simulink model "CSI_0313_4DC"  (R2018a)
settings: Solver=FixedStepDiscrete  StartTime=0.0  StopTime=Tstop  FixedStep=Tdelt  MaxStep=1e-4  RelTol=1e-3
values from neighbouring files (symbols this model uses):
  C = 12e-6    (= 1.2e-05)    [Inputparameter.m]
  Cdc = 4.76*10^-3    (= 0.00476)    [Inputparameter.m]
  Cemc = 1.5e-6    (= 1.5e-06)    [Inputparameter.m]
  fanalog = 7000    [Run.m]
  fKIUdc = 6    [Run.m]
  fKPUdc = 0.4    [Run.m]
  fTs = Update/18000    (= 0.000111111111111)    [Run.m]
  K120 = 0.0    (= 0)    [Run.m]
  K21 = 0.0    (= 0)    [Run.m]
  K5 = 0.0    (= 0)    [Run.m]
  K7 = 0.0    (= 0)    [Run.m]
  Kipll = 1.0    (= 1)    [Run.m]
  klmt = 0.3    [Run.m]
  Kpll = 20.0    (= 20)    [Run.m]
  Lgrid = 7.717e-4*10    (= 0.007717)    [Run.m]
  Lline = 60e-6    (= 6e-05)    [Inputparameter.m]
  Lpwm = 184.8e-6    (= 0.0001848)    [Inputparameter.m]
  mode = 1    [Run.m]
  Nsw = 18000/fbase    [Run.m]
  Qbpf = 1.0    (= 1)    [Run.m]
  Rc = 10e-3    (= 0.01)    [Inputparameter.m]
  Remc = 1e-3    (= 0.001)    [Inputparameter.m]
  Rgrid = 2*pi*fbase*Lgrid/XR    [Run.m]
  Rline = 4.95e-3    (= 0.00495)    [Inputparameter.m]
  Rpre = 2.2    [Inputparameter.m]
  Rpwm = 6.2e-3    (= 0.0062)    [Inputparameter.m]
  Tdelt = (fTs)/(200*Update)    (= 2.77777777778e-07)    [Run.m]
  Tdt = 1.27e-6    (= 1.27e-06)    [Run.m]
  tstart = 0.2    [Run.m]
  Tvstep = 1.5    [Run.m]
  Update = 2    [Run.m]
  Vbase = 400*sqrt(2/3)    [Inputparameter.m]
undefined symbols (not defined in the file or in its folder): sigbuilder_block
libraries: powerlib x412
(part 12 of 13)

== matlab function CSI_0313_4DC/AIP6/Subsystem5/PLL/Pos&Neg seq extract in subsystem /IIR_BPF_Re1 ==
  data: u input; fn input; fQ parameter; y output; fTs parameter; iMode parameter
function y =IIR_2rd(u, fn, fQ, fTs, iMode)
    % Second order transfer function used for LPF and BPF
    % y[n] = (fa1*x[n]+fa2*x[n-1]+fa3*x[n-2]-fb2*y[n-1]-fb3*y[n-2])/fb1
    % u:  error input
    % fn:  Natural frequency
    % fQ:   Quality factor
    % fTs:  Sampling time
    % iMode: Mode Selection
    % iMode=1 used as generalized 2nd-order LPF, LPF(s)=wn^2/(s^2+wn/Q*s+wn^2)
    % iMode=2 used as 2nd-order LPF in SOGI, SOGI_LPF(s)=(wn^2/Q)/(s^2+wn/Q*s+wn^2)
    % iMode=3 used as 2nd-order BPF in SOGI, SOGI_BPF(s)=(wn*s/Q)/(s^2+wn/Q*s+wn^2)
    
    persistent t;
    
    if isempty(t)
        t = zeros(2,3);
    end
    
    wn = 2*pi*fn;
    wc = wn/fQ;

    fT1 = wc*wn*fTs*fTs; 
    fT2 = 2*wc*fTs;
    fT3 = (wn*fTs)^2;
    
    fb1 = fT3+fT2+4;
    fb2 = 2*fT3-8;
    fb3 = fT3-fT2+4;
    
    if (iMode ==1)
        fa1 = fT3;
        fa2 = 2*fT3;
        fa3 = fT3;
    elseif (iMode ==2)
        fa1 = fT1;
        fa2 = 2*fT1;
        fa3 = fT1;
    else
        fa1 = fT2;
        fa2 = 0;
        fa3 = -fT2;
    end
%     if(Trigs > 0)
        t(1,1) = u;        
        t(2,1) = (fa1*t(1,1)+fa2*t(1,2)+fa3*t(1,3)-fb2*t(2,2)-fb3*t(2,3))/fb1;
    
        t(1,3) = t(1,2);
        t(1,2) = t(1,1);
        
        t(2,3) = t(2,2);
        t(2,2) = t(2,1);
%     else
%         t(1,1) = t(1,1);        
%         t(2,1) = t(2,1);
%     
%         t(1,3) = t(1,3);
%         t(1,2) = t(1,2);
%         
%         t(2,3) = t(2,3);
%         t(2,2) = t(2,2);
%     end
    
    y = t(2,1);    
end

== matlab function CSI_0313_4DC/AIP6/Subsystem5/PLL/Pos&Neg seq extract in subsystem /IIR_LPF_Im ==
  data: u input; fn input; fQ parameter; y output; fTs parameter; iMode parameter
function y =IIR_2rd(u, fn, fQ, fTs, iMode)
    % Second order transfer function used for LPF and BPF
    % y[n] = (fa1*x[n]+fa2*x[n-1]+fa3*x[n-2]-fb2*y[n-1]-fb3*y[n-2])/fb1
    % u:  error input
    % fn:  Natural frequency
    % fQ:   Quality factor
    % fTs:  Sampling time
    % iMode: Mode Selection
    % iMode=1 used as generalized 2nd-order LPF, LPF(s)=wn^2/(s^2+wn/Q*s+wn^2)
    % iMode=2 used as 2nd-order LPF in SOGI, SOGI_LPF(s)=(wn^2/Q)/(s^2+wn/Q*s+wn^2)
    % iMode=3 used as 2nd-order BPF in SOGI, SOGI_BPF(s)=(wn*s/Q)/(s^2+wn/Q*s+wn^2)
    
    persistent t;
    
    if isempty(t)
        t = zeros(2,3);
    end
    
    wn = 2*pi*fn;
    wc = wn/fQ;

    fT1 = wc*wn*fTs*fTs; 
    fT2 = 2*wc*fTs;
    fT3 = (wn*fTs)^2;
    
    fb1 = fT3+fT2+4;
    fb2 = 2*fT3-8;
    fb3 = fT3-fT2+4;
    
    if (iMode ==1)
        fa1 = fT3;
        fa2 = 2*fT3;
        fa3 = fT3;
    elseif (iMode ==2)
        fa1 = fT1;
        fa2 = 2*fT1;
        fa3 = fT1;
    else
        fa1 = fT2;
        fa2 = 0;
        fa3 = -fT2;
    end
        
%    if(Trigs > 0)
        t(1,1) = u;        
        t(2,1) = (fa1*t(1,1)+fa2*t(1,2)+fa3*t(1,3)-fb2*t(2,2)-fb3*t(2,3))/fb1;
    
        t(1,3) = t(1,2);
        t(1,2) = t(1,1);
        
        t(2,3) = t(2,2);
        t(2,2) = t(2,1);
%     else
%         t(1,1) = t(1,1);        
%         t(2,1) = t(2,1);
%     
%         t(1,3) = t(1,3);
%         t(1,2) = t(1,2);
%         
%         t(2,3) = t(2,3);
%         t(2,2) = t(2,2);
%     end
%     
    y = t(2,1);    
end

== matlab function CSI_0313_4DC/AIP6/Subsystem5/PLL/Pos&Neg seq extract in subsystem /IIR_LPF_Re1 ==
  data: u input; fn input; fQ parameter; y output; fTs parameter; iMode parameter
function y =IIR_2rd(u, fn, fQ, fTs, iMode)
    % Second order transfer function used for LPF and BPF
    % y[n] = (fa1*x[n]+fa2*x[n-1]+fa3*x[n-2]-fb2*y[n-1]-fb3*y[n-2])/fb1
    % u:  error input
    % fn:  Natural frequency
    % fQ:   Quality factor
    % fTs:  Sampling time
    % iMode: Mode Selection
    % iMode=1 used as generalized 2nd-order LPF, LPF(s)=wn^2/(s^2+wn/Q*s+wn^2)
    % iMode=2 used as 2nd-order LPF in SOGI, SOGI_LPF(s)=(wn^2/Q)/(s^2+wn/Q*s+wn^2)
    % iMode=3 used as 2nd-order BPF in SOGI, SOGI_BPF(s)=(wn*s/Q)/(s^2+wn/Q*s+wn^2)
    
    persistent t;
    
    if isempty(t)
        t = zeros(2,3);
    end
    
    wn = 2*pi*fn;
    wc = wn/fQ;

    fT1 = wc*wn*fTs*fTs; 
    fT2 = 2*wc*fTs;
    fT3 = (wn*fTs)^2;
    
    fb1 = fT3+fT2+4;
    fb2 = 2*fT3-8;
    fb3 = fT3-fT2+4;
    
    if (iMode ==1)
        fa1 = fT3;
        fa2 = 2*fT3;
        fa3 = fT3;
    elseif (iMode ==2)
        fa1 = fT1;
        fa2 = 2*fT1;
        fa3 = fT1;
    else
        fa1 = fT2;
        fa2 = 0;
        fa3 = -fT2;
    end
        
%    if(Trigs > 0)
        t(1,1) = u;        
        t(2,1) = (fa1*t(1,1)+fa2*t(1,2)+fa3*t(1,3)-fb2*t(2,2)-fb3*t(2,3))/fb1;
    
        t(1,3) = t(1,2);
        t(1,2) = t(1,1);
        
        t(2,3) = t(2,2);
        t(2,2) = t(2,1);
%     else
%         t(1,1) = t(1,1);        
%         t(2,1) = t(2,1);
%     
%         t(1,3) = t(1,3);
%         t(1,2) = t(1,2);
%         
%         t(2,3) = t(2,3);
%         t(2,2) = t(2,2);
%     end
    
    y = t(2,1);    
end

== matlab function CSI_0313_4DC/AIP6/Subsystem5/PLL/RIZ_To_DQ0 ==
  data: RIZ input; DQ0 output; wt input; iAxis parameter
function DQ0 = RIZ_To_DQ0(RIZ,wt,iAxis)
    % Park Transfer from Re-Im axis to DQ0 axis
    DQ0 = [0;0;0];
    if (iAxis == 1)
        DQ0(1) = RIZ(1)*cos(wt)+RIZ(2)*sin(wt);
        DQ0(2) = -RIZ(1)*sin(wt)+RIZ(2)*cos(wt);
    else
        DQ0(1) = RIZ(1)*sin(wt)-RIZ(2)*cos(wt);
        DQ0(2) = RIZ(1)*cos(wt)+RIZ(2)*sin(wt);
    end
end

== matlab function CSI_0313_4DC/AIP6/Subsystem7/ABC_To_RIZ1 ==
  data: ABC input; RIZ output
function RIZ = ABC_To_RIZ(ABC)
    % Clarke Transfer from ABC axis to Re-Im axis
    RIZ = [0;0;0];
    RIZ(1) = (2*ABC(1)-ABC(2)-ABC(3))/3;
    RIZ(2) = sqrt(3)*(ABC(2)-ABC(3))/3;
    RIZ(3) = (ABC(1)+ABC(2)+ABC(3))/3;
end

== matlab function CSI_0313_4DC/AIP6/Subsystem7/BPF /IIR_BPF_Re1 ==
  data: u input; fn input; fQ parameter; y output; fTs parameter; iMode parameter
function y =IIR_2rd(u, fn, fQ, fTs, iMode)
    % Second order transfer function used for LPF and BPF
    % y[n] = (fa1*x[n]+fa2*x[n-1]+fa3*x[n-2]-fb2*y[n-1]-fb3*y[n-2])/fb1
    % u:  error input
    % fn:  Natural frequency
    % fQ:   Quality factor
    % fTs:  Sampling time
    % iMode: Mode Selection
    % iMode=1 used as generalized 2nd-order LPF, LPF(s)=wn^2/(s^2+wn/Q*s+wn^2)
    % iMode=2 used as 2nd-order LPF in SOGI, SOGI_LPF(s)=(wn^2/Q)/(s^2+wn/Q*s+wn^2)
    % iMode=3 used as 2nd-order BPF in SOGI, SOGI_BPF(s)=(wn*s/Q)/(s^2+wn/Q*s+wn^2)
    
    persistent t;
    
    if isempty(t)
        t = zeros(2,3);
    end
    
    wn = 2*pi*fn;
    wc = wn/fQ;

    fT1 = wc*wn*fTs*fTs; 
    fT2 = 2*wc*fTs;
    fT3 = (wn*fTs)^2;
    
    fb1 = fT3+fT2+4;
    fb2 = 2*fT3-8;
    fb3 = fT3-fT2+4;
    
    if (iMode ==1)
        fa1 = fT3;
        fa2 = 2*fT3;
        fa3 = fT3;
    elseif (iMode ==2)
        fa1 = fT1;
        fa2 = 2*fT1;
        fa3 = fT1;
    else
        fa1 = fT2;
        fa2 = 0;
        fa3 = -fT2;
    end
 
        t(1,1) = u;        
        t(2,1) = (fa1*t(1,1)+fa2*t(1,2)+fa3*t(1,3)-fb2*t(2,2)-fb3*t(2,3))/fb1;
    
        t(1,3) = t(1,2);
        t(1,2) = t(1,1);
        
        t(2,3) = t(2,2);
        t(2,2) = t(2,1);
 
    
    y = t(2,1);    
end

== matlab function CSI_0313_4DC/AIP6/Subsystem7/BPF /IIR_BPF_Re2 ==
  data: u input; fn input; fQ parameter; y output; fTs parameter; iMode parameter
function y =IIR_2rd(u, fn, fQ, fTs, iMode)
    % Second order transfer function used for LPF and BPF
    % y[n] = (fa1*x[n]+fa2*x[n-1]+fa3*x[n-2]-fb2*y[n-1]-fb3*y[n-2])/fb1
    % u:  error input
    % fn:  Natural frequency
    % fQ:   Quality factor
    % fTs:  Sampling time
    % iMode: Mode Selection
    % iMode=1 used as generalized 2nd-order LPF, LPF(s)=wn^2/(s^2+wn/Q*s+wn^2)
    % iMode=2 used as 2nd-order LPF in SOGI, SOGI_LPF(s)=(wn^2/Q)/(s^2+wn/Q*s+wn^2)
    % iMode=3 used as 2nd-order BPF in SOGI, SOGI_BPF(s)=(wn*s/Q)/(s^2+wn/Q*s+wn^2)
    
    persistent t;
    
    if isempty(t)
        t = zeros(2,3);
    end
    
    wn = 2*pi*fn;
    wc = wn/fQ;

    fT1 = wc*wn*fTs*fTs; 
    fT2 = 2*wc*fTs;
    fT3 = (wn*fTs)^2;
    
    fb1 = fT3+fT2+4;
    fb2 = 2*fT3-8;
    fb3 = fT3-fT2+4;
    
    if (iMode ==1)
        fa1 = fT3;
        fa2 = 2*fT3;
        fa3 = fT3;
    elseif (iMode ==2)
        fa1 = fT1;
        fa2 = 2*fT1;
        fa3 = fT1;
    else
        fa1 = fT2;
        fa2 = 0;
        fa3 = -fT2;
    end
  
        t(1,1) = u;        
        t(2,1) = (fa1*t(1,1)+fa2*t(1,2)+fa3*t(1,3)-fb2*t(2,2)-fb3*t(2,3))/fb1;
    
        t(1,3) = t(1,2);
        t(1,2) = t(1,1);
        
        t(2,3) = t(2,2);
        t(2,2) = t(2,1);
 
    
    y = t(2,1);    
end

== matlab function CSI_0313_4DC/AIP6/Subsystem7/BPF /IIR_BPF_Re3 ==
  data: u input; fn input; fQ parameter; y output; fTs parameter; iMode parameter
function y =IIR_2rd(u, fn, fQ, fTs, iMode)
    % Second order transfer function used for LPF and BPF
    % y[n] = (fa1*x[n]+fa2*x[n-1]+fa3*x[n-2]-fb2*y[n-1]-fb3*y[n-2])/fb1
    % u:  error input
    % fn:  Natural frequency
    % fQ:   Quality factor
    % fTs:  Sampling time
    % iMode: Mode Selection
    % iMode=1 used as generalized 2nd-order LPF, LPF(s)=wn^2/(s^2+wn/Q*s+wn^2)
    % iMode=2 used as 2nd-order LPF in SOGI, SOGI_LPF(s)=(wn^2/Q)/(s^2+wn/Q*s+wn^2)
    % iMode=3 used as 2nd-order BPF in SOGI, SOGI_BPF(s)=(wn*s/Q)/(s^2+wn/Q*s+wn^2)
    
    persistent t;
    
    if isempty(t)
        t = zeros(2,3);
    end
    
    wn = 2*pi*fn;
    wc = wn/fQ;

    fT1 = wc*wn*fTs*fTs; 
    fT2 = 2*wc*fTs;
    fT3 = (wn*fTs)^2;
    
    fb1 = fT3+fT2+4;
    fb2 = 2*fT3-8;
    fb3 = fT3-fT2+4;
    
    if (iMode ==1)
        fa1 = fT3;
        fa2 = 2*fT3;
        fa3 = fT3;
    elseif (iMode ==2)
        fa1 = fT1;
        fa2 = 2*fT1;
        fa3 = fT1;
    else
        fa1 = fT2;
        fa2 = 0;
        fa3 = -fT2;
    end
  
        t(1,1) = u;        
        t(2,1) = (fa1*t(1,1)+fa2*t(1,2)+fa3*t(1,3)-fb2*t(2,2)-fb3*t(2,3))/fb1;
    
        t(1,3) = t(1,2);
        t(1,2) = t(1,1);
        
        t(2,3) = t(2,2);
        t(2,2) = t(2,1);
 
    
    y = t(2,1);    
end

== matlab function CSI_0313_4DC/AIP6/Subsystem7/Pos Compensation1/DQ0_To_RIZ ==
  data: DQ0 input; RIZ output; wt input; iAxis parameter
function RIZ = DQ0_To_RIZ(DQ0,wt,iAxis)
    % Inverse Park Transfer from DQ0 axis to Re-Im axis
    RIZ = [0;0;0];
    if (iAxis == 1)
        RIZ(1) = DQ0(1)*cos(wt)-DQ0(2)*sin(wt);
        RIZ(2) = DQ0(1)*sin(wt)+DQ0(2)*cos(wt);
    else
        RIZ(1) = DQ0(1)*sin(wt)+DQ0(2)*cos(wt);
        RIZ(2) = -DQ0(1)*cos(wt)+DQ0(2)*sin(wt);
    end
end

== matlab function CSI_0313_4DC/AIP10/Subsystem3/IIR_1st1 ==
  data: u input; fc parameter; y output; fTs parameter
function y = IIR_1st(u, fc, fTs)
    % y[n] = (-(1-T)*y[n-1] + x[n] + x[n-1])/(1+T)
    % u:    Input
    % fc:   Cut-off frequency
    % fTs:  Sample time
    
    persistent t;
    
    if isempty(t)
        t = zeros(2,2);
    end
    
    T = 1/(pi*fc*fTs);            
    
%     if(Trig > 0)
        t(1,1) = u;        
        t(2,1) = (t(1,1) + t(1,2) - (1-T)*t(2,2)) / (1+T);
    
        t(1,2) = t(1,1);
        t(2,2) = t(2,1);
%     else
%         t(1,1) = t(1,1);        
%         t(2,1) = t(2,1);
%     
%         t(1,2) = t(1,2);
%         t(2,2) = t(2,2);
%     end
%     
    y = t(2,1);
end

== matlab function CSI_0313_4DC/AIP6/Subsystem7/Pos Compensation1/RIZ_To_ABC ==
  data: RIZ input; ABC output
function ABC = RIZ_To_ABC(RIZ)
    % Inverse Clarke Transfer from Re-Im axis to ABC axis
    ABC = [0;0;0];
    ABC(1) = RIZ(1)+RIZ(3);
    ABC(2) = -(RIZ(1)-sqrt(3)*RIZ(2))/2+RIZ(3);
    ABC(3) = -(RIZ(1)+sqrt(3)*RIZ(2))/2+RIZ(3);
end

== matlab function CSI_0313_4DC/AIP6/Subsystem7/Pos Compensation1/RIZ_To_DQ0 ==
  data: RIZ input; DQ0 output; wt input; iAxis parameter
function DQ0 = RIZ_To_DQ0(RIZ,wt,iAxis)
    % Park Transfer from Re-Im axis to DQ0 axis
    DQ0 = [0;0;0];
    if (iAxis == 1)
        DQ0(1) = RIZ(1)*cos(wt)+RIZ(2)*sin(wt);
        DQ0(2) = -RIZ(1)*sin(wt)+RIZ(2)*cos(wt);
    else
        DQ0(1) = RIZ(1)*sin(wt)-RIZ(2)*cos(wt);
        DQ0(2) = RIZ(1)*cos(wt)+RIZ(2)*sin(wt);
    end
end

== matlab function CSI_0313_4DC/AIP6/Subsystem7/RIZ_To_ABC1 ==
  data: RIZ input; ABC output
function ABC = RIZ_To_ABC(RIZ)
    % Inverse Clarke Transfer from Re-Im axis to ABC axis
    ABC = [0;0;0];
    ABC(1) = RIZ(1)+RIZ(3);
    ABC(2) = -(RIZ(1)-sqrt(3)*RIZ(2))/2+RIZ(3);
    ABC(3) = -(RIZ(1)+sqrt(3)*RIZ(2))/2+RIZ(3);
end

== matlab function CSI_0313_4DC/AIP6/Subsystem7/Subsystem5/3rd Injection1 ==
  data: Vabc input; Mod output size=3; Vdc input; mode parameter
function Mod = fcn(Vabc,Vdc,mode)

Mod = Vabc./(Vdc/2);
Vmin = min(Mod(1),min(Mod(2),Mod(3)));
Vmax = max(Mod(1),max(Mod(2),Mod(3)));
Vinj= -0.5*(Vmin+Vmax);
if(mode == 0)
    Mod(1) = Mod(1)+Vinj;
    Mod(2) = Mod(2)+Vinj;
    Mod(3) = Mod(3)+Vinj;
else
    Mod(1) = Mod(1);
    Mod(2) = Mod(2);
    Mod(3) = Mod(3);    
end
end

function y = min(a,b)
    if (a <= b)
        y = a;
    else
        y = b;
    end
end

function y = max(a,b)
    if (a >= b)
        y = a;
    else
        y = b;
    end
end

== matlab function CSI_0313_4DC/AIP6/VLine_To_VPh ==
  data: VLine input; VPh output
function VPh = VLine_To_VPh(VLine)
    % Assume Van+Vbn+Vcn=0
    % VLine(1)=Vab; VLine(2)=Vbc; VLine(3)=Vca 
    % VPh(1)=Van; VPh(2)=Vbn; VPh(3)=Vcn;
    VPh = [0;0;0];
    VPh(1) = (VLine(1)-VLine(3))/3;
    VPh(2) = (VLine(2)-VLine(1))/3;
    VPh(3) = (VLine(3)-VLine(2))/3;
end

== matlab function CSI_0313_4DC/AIP8/Moving average ==
  data: yout output; uin input; trig input; iNumAvg parameter; iNumDly parameter; ubase parameter
function yout=sample(uin,trig,iNumAvg,iNumDly,ubase)

persistent uary cnt sum yavg;

iNumIn = length(uin);
iNumDly = iNumDly+1;
if isempty(cnt)  
    cnt = 0;
    uary = zeros(iNumIn,iNumAvg);
    sum = zeros(iNumIn,1);
    yavg = zeros(iNumIn,iNumDly);   
end

if(trig >0) 
    for i=1:1:iNumIn
        for j=iNumDly:-1:2
            yavg(i,j)= yavg(i,j-1);
        end
    end
    cnt = cnt +1;
    for i=1:1:iNumIn
         uary(i,cnt) = uin(i)/ubase;            
        for j=1:1:iNumAvg
        sum(i) = sum(i)+uary(i,j);
        end
    end
       for i=1:1:iNumIn
            yavg(i,1)=sum(i)/iNumAvg;
       end
        
        for i=1:1:iNumIn
            sum(i)=0;
        end
        if(cnt >= iNumAvg)
            cnt = 0;
        end
end
    yout = yavg(:,iNumDly);
end

== matlab function CSI_0313_4DC/AIP10/Subsystem5/PLL/ABC_To_RIZ ==
  data: ABC input size=3; RIZ output size=3
function RIZ = ABC_To_RIZ(ABC)
    % Clarke Transfer from ABC axis to Re-Im axis
    RIZ = [0;0;0];
    RIZ(1) = (2*ABC(1)-ABC(2)-ABC(3))/3;
    RIZ(2) = sqrt(3)*(ABC(2)-ABC(3))/3;
    RIZ(3) = (ABC(1)+ABC(2)+ABC(3))/3;
end

== matlab function CSI_0313_4DC/AIP8/SPWM_Three Level/Carrier Gen ==
  data: carrier output; sgn output; fdelt parameter; fsw input size=1
function [carrier, sgn] = fcn(fdelt, fsw)

persistent waveSaw stage;
if isempty(waveSaw)
    waveSaw = 0;
    stage = 0;
end

fHtop = 1/fdelt;
fHalf = 0.5*fHtop;
if (waveSaw < fHalf)
    waveTri = waveSaw;
else
    waveTri = fHtop - waveSaw;
end
sgn = 1-stage;
if (waveSaw < (fHalf-0.5*fsw))
    stage = 1;
elseif (waveSaw < (fHtop-0.5*fsw))
    sgn = stage;
    stage = 0;
else
	stage = 1;
end
	waveSaw = waveSaw + fsw;
if (waveSaw >= fHtop)
    waveSaw = waveSaw - fHtop;
end

carrier = waveTri / fHalf;

end

== matlab function CSI_0313_4DC/AIP8/SPWM_Three Level/Pulse Modulation ==
  data: carrier input; Pulse output; sgn input; update input; mod input; chk output; chk1 output
function [Pulse,chk,chk1] = fcn(carrier, sgn, update, mod)

persistent intx cnt;
if isempty(intx)
    intx = zeros(3,1);
    ref = zeros(3,1);    
    cnt = zeros(3,1);
end

Gate = zeros(3,4);
carrier_up = carrier;
carrier_down = carrier-1;

for i=1:1:3
    if(update > 0)
        ref(i) = mod(i);
        cnt(i) = 0;
    else
        ref(i) = intx(i);        
    end    
    intx(i) = ref(i);
    %Limitter
    if(ref(i) > 0.99)   
        ref(i) = 0.99;
    elseif(ref(i) < -0.99)
        ref(i) = -0.99;
    end
%%%%%%%%%%%    
end

for i=1:1:3
    if (ref(i) >= carrier_up)
       Gate(i,1) = 1;
       Gate(i,3) = 0;
    elseif (ref(i) <= carrier_up)
       Gate(i,1) = 0;
       Gate(i,3) = 1;
    end
    
    if (ref(i) >= carrier_down)
       Gate(i,2) = 1;
       Gate(i,4) = 0;
    elseif (ref(i) <= carrier_down)
       Gate(i,2) = 0;
       Gate(i,4) = 1;
    end
end
 
Pulse = [Gate(1,:), Gate(2,:),Gate(3,:)];
chk = Gate(1,:) ;
chk1 = ref(1) ;

end

== matlab function CSI_0313_4DC/AIP8/SPWM_Three Level/Tdt Insert ==
  data: Gate output; pulse input; tdt parameter; fdelt parameter; st input; chk output
function [Gate, chk] = fcn(pulse, tdt, fdelt, st)

persistent intx cnt;
if isempty(intx)
    intx = zeros(12,1);
    cnt = zeros(12,1);
end
Gate = pulse;

for i=1:1:12
    if( (Gate(i)==1) && (intx(i)==0) )
			cnt(i) = cnt(i)+fdelt;
			if (cnt(i) >= tdt)
				Gate(i) = 1;
				intx(i) = 1;
				cnt(i) = 0;
			else
				Gate(i) = intx(i);
            end
    else
			intx(i) = Gate(i);
			cnt(i)  = 0;
    end
    if(st == 0)
    	Gate(i) = 0;
    end
end
chk = Gate;

end

== matlab function CSI_0313_4DC/AIP8/SPWM_Three Level/Voltage update timing generator ==
  data: Trigger input; Tupdate output; Update input
function Tupdate = fcn(Trigger,Update)
    persistent cntx Tupdate1;
    if isempty(cntx)
        cntx = 2*Update-1;
        Tupdate1 = 0;
    end
    
    if(Trigger > 0)
        cntx = cntx +1;
    else
        cntx = cntx;
    end
    
    
    if(Trigger > 0 && cntx == 4)
        Tupdate1 = Trigger;
    else
        Tupdate1 = 0;        
    end
    if(cntx == 2*Update)
        cntx = 0;
    end

    Tupdate = Tupdate1;

== matlab function CSI_0313_4DC/AIP8/SPWM_Three Level/Voltage update timing generator1 ==
  data: Trigger input; Tupdate output; Update input
function Tupdate = fcn(Trigger,Update)
    persistent cntx Tupdate1;
    if isempty(cntx)
         if(Update == 1)
            cntx =  1;
         else
            cntx =  3;
         end
        Tupdate1 = 0;
    end
    
    if(Trigger > 0)
        cntx = cntx +1;
    else
        cntx = cntx;
    end
    
    
    if(Trigger > 0 && cntx == 2)
        Tupdate1 = Trigger;
    else
        Tupdate1 = 0;        
    end
    if(cntx == 2*Update)
        cntx = 0;
    end

    Tupdate = Tupdate1;

== matlab function CSI_0313_4DC/AIP8/Sample//Moving window5 ==
  data: yout output; uin input; trig input; iNumAvg parameter; iNumDly parameter; ubase parameter
function yout=sample(uin,trig,iNumAvg,iNumDly,ubase)

persistent uary cnt sum yavg;

iNumIn = length(uin);
iNumDly = iNumDly+1;
if isempty(cnt)  
    cnt = 0;
    uary = zeros(iNumIn,iNumAvg);
    sum = zeros(iNumIn,1);
    yavg = zeros(iNumIn,iNumDly);    
end

if(trig >0) 
    for i=1:1:iNumIn
        for j=iNumDly:-1:2
            yavg(i,j)= yavg(i,j-1);
        end
    end
    cnt = cnt +1;
    for i=1:1:iNumIn
        uary(i,cnt) = uin(i)/ubase;
        sum(i) = sum(i)+uary(i,cnt);
    end
    if(cnt == iNumAvg)
        cnt = 0;
        for i=1:1:iNumIn
            yavg(i,1)=sum(i)/iNumAvg;
        end
        for i=1:1:iNumIn
            sum(i)=0;
        end
    end        
end
    yout = yavg(:,iNumDly);
end

== matlab function CSI_0313_4DC/AIP8/Subsystem/IIR_1st1 ==
  data: u input; fc parameter; y output; fTs parameter
function y = IIR_1st(u, fc, fTs)
    % y[n] = (-(1-T)*y[n-1] + x[n] + x[n-1])/(1+T)
    % u:    Input
    % fc:   Cut-off frequency
    % fTs:  Sample time
    
    persistent t;
    
    if isempty(t)
        t = zeros(2,2);
    end
    
    T = 1/(pi*fc*fTs);            
    
%     if(Trig > 0)
        t(1,1) = u;        
        t(2,1) = (t(1,1) + t(1,2) - (1-T)*t(2,2)) / (1+T);
    
        t(1,2) = t(1,1);
        t(2,2) = t(2,1);
%     else
%         t(1,1) = t(1,1);        
%         t(2,1) = t(2,1);
%     
%         t(1,2) = t(1,2);
%         t(2,2) = t(2,2);
%     end
%     
    y = t(2,1);
end

== matlab function CSI_0313_4DC/AIP8/Subsystem/IIR_1st2 ==
  data: u input; fc parameter; y output; fTs parameter
function y = IIR_1st(u, fc, fTs)
    % y[n] = (-(1-T)*y[n-1] + x[n] + x[n-1])/(1+T)
    % u:    Input
    % fc:   Cut-off frequency
    % fTs:  Sample time
    
    persistent t;
    
    if isempty(t)
        t = zeros(2,2);
    end
    
    T = 1/(pi*fc*fTs);            
    
%     if(Trig > 0)
        t(1,1) = u;        
        t(2,1) = (t(1,1) + t(1,2) - (1-T)*t(2,2)) / (1+T);
    
        t(1,2) = t(1,1);
        t(2,2) = t(2,1);
%     else
%         t(1,1) = t(1,1);        
%         t(2,1) = t(2,1);
%     
%         t(1,2) = t(1,2);
%         t(2,2) = t(2,2);
%     end
%     
    y = t(2,1);
end

== matlab function CSI_0313_4DC/AIP8/Subsystem/IIR_1st3 ==
  data: u input; fc parameter; y output; fTs parameter
function y = IIR_1st(u, fc, fTs)
    % y[n] = (-(1-T)*y[n-1] + x[n] + x[n-1])/(1+T)
    % u:    Input
    % fc:   Cut-off frequency
    % fTs:  Sample time
    
    persistent t;
    
    if isempty(t)
        t = zeros(2,2);
    end
    
    T = 1/(pi*fc*fTs);            
    
%     if(Trig > 0)
        t(1,1) = u;        
        t(2,1) = (t(1,1) + t(1,2) - (1-T)*t(2,2)) / (1+T);
    
        t(1,2) = t(1,1);
        t(2,2) = t(2,1);
%     else
%         t(1,1) = t(1,1);        
%         t(2,1) = t(2,1);
%     
%         t(1,2) = t(1,2);
%         t(2,2) = t(2,2);
%     end
%     
    y = t(2,1);
end

== matlab function CSI_0313_4DC/AIP10/Subsystem5/PLL/Integral ==
  data: u input; fGain parameter; fTs parameter; y output
function y  = Integral(u, fGain, fTs)
    % y[n] = y[n-1] + (TS*0.5)*(x[n]+x[n-1])
    % u:     input
    % fGain: Gain
    % fTs:  Sampling time
    
    % t(1,2) stores x[n],x[n-1]; t(2,2) stores y[n],y[n-1]
    persistent t;      
    if isempty(t)           % Initialization
        t = zeros(2,2);
    end
%     if(Trig > 0)
        t(1,1) = u;
        t(2,1) = t(2,2) + fGain*0.5*fTs*(t(1,1)+t(1,2));   

        t(1,2) = t(1,1);
        t(2,2) = t(2,1);
%     else
%         t(1,1) = t(1,1);
%         t(2,1) = t(2,1);   
% 
%         t(1,2) = t(1,2);
%         t(2,2) = t(2,2);
%     end
    y = t(2,1);
end

== matlab function CSI_0313_4DC/AIP10/Subsystem5/PLL/PI Ctrl ==
  data: err input; y output; fKI parameter; fMinLmt parameter; fTs parameter; fMaxLmt parameter; fKP parameter
function y = PICtrl(err, fKI, fMinLmt, fTs, fMaxLmt, fKP)
    % y[n] = y[n-1] + KP*(x[n]-x[n-1]) + (KP*KI*TS*0.5)*(x[n]+x[n-1])
    % err:  error input
    % fKP:   Proportional gain
    % fKI:   Integral Coefficient
    % fMinLmt: Minimum limitation
    % fMaxLmt: Maximum limitation
    % fTs:  Sampling time
    
    % t(1,2) stores x[n],x[n-1]; t(2,2) stores y[n],y[n-1]
    persistent t;      
    if isempty(t)           % Initialization
        t = zeros(2,2);
    end

%     if(Trig > 0)
        t(1,1) = err;
        t(2,1) = t(2,2) + fKP*(t(1,1)-t(1,2)) + fKP*fKI*0.5*(t(1,1)+t(1,2))*fTs;   
    
        if (t(2,1) < fMinLmt)
            t(2,1) = fMinLmt;
        elseif (t(2,1) > fMaxLmt)
            t(2,1) = fMaxLmt;
        end
        t(1,2) = t(1,1);
        t(2,2) = t(2,1);
%     else
%         t(1,1) = t(1,1);
%         t(2,1) = t(2,1);   
%         t(1,2) = t(1,2);
%         t(2,2) = t(2,2);
%     end
    
    y = t(2,1);
end

== matlab function CSI_0313_4DC/AIP10/Subsystem5/PLL/Pos&Neg seq extract in subsystem /IIR_BPF_Im ==
  data: u input; fn input; fQ parameter; y output; fTs parameter; iMode parameter
function y =IIR_2rd(u, fn, fQ, fTs, iMode)
    % Second order transfer function used for LPF and BPF
    % y[n] = (fa1*x[n]+fa2*x[n-1]+fa3*x[n-2]-fb2*y[n-1]-fb3*y[n-2])/fb1
    % u:  error input
    % fn:  Natural frequency
    % fQ:   Quality factor
    % fTs:  Sampling time
    % iMode: Mode Selection
    % iMode=1 used as generalized 2nd-order LPF, LPF(s)=wn^2/(s^2+wn/Q*s+wn^2)
    % iMode=2 used as 2nd-order LPF in SOGI, SOGI_LPF(s)=(wn^2/Q)/(s^2+wn/Q*s+wn^2)
    % iMode=3 used as 2nd-order BPF in SOGI, SOGI_BPF(s)=(wn*s/Q)/(s^2+wn/Q*s+wn^2)
    
    persistent t;
    
    if isempty(t)
        t = zeros(2,3);
    end
    
    wn = 2*pi*fn;
    wc = wn/fQ;

    fT1 = wc*wn*fTs*fTs; 
    fT2 = 2*wc*fTs;
    fT3 = (wn*fTs)^2;
    
    fb1 = fT3+fT2+4;
    fb2 = 2*fT3-8;
    fb3 = fT3-fT2+4;
    
    if (iMode ==1)
        fa1 = fT3;
        fa2 = 2*fT3;
        fa3 = fT3;
    elseif (iMode ==2)
        fa1 = fT1;
        fa2 = 2*fT1;
        fa3 = fT1;
    else
        fa1 = fT2;
        fa2 = 0;
        fa3 = -fT2;
    end
        
%     if(Trigs > 0)
        t(1,1) = u;        
        t(2,1) = (fa1*t(1,1)+fa2*t(1,2)+fa3*t(1,3)-fb2*t(2,2)-fb3*t(2,3))/fb1;
    
        t(1,3) = t(1,2);
        t(1,2) = t(1,1);
        
        t(2,3) = t(2,2);
        t(2,2) = t(2,1);
%     else
%         t(1,1) = t(1,1);        
%         t(2,1) = t(2,1);
%     
%         t(1,3) = t(1,3);
%         t(1,2) = t(1,2);
%         
%         t(2,3) = t(2,3);
%         t(2,2) = t(2,2);
%     end
    
    y = t(2,1);    
end

== matlab function CSI_0313_4DC/AIP10/Subsystem5/PLL/Pos&Neg seq extract in subsystem /IIR_BPF_Re1 ==
  data: u input; fn input; fQ parameter; y output; fTs parameter; iMode parameter
function y =IIR_2rd(u, fn, fQ, fTs, iMode)
    % Second order transfer function used for LPF and BPF
    % y[n] = (fa1*x[n]+fa2*x[n-1]+fa3*x[n-2]-fb2*y[n-1]-fb3*y[n-2])/fb1
    % u:  error input
    % fn:  Natural frequency
    % fQ:   Quality factor
    % fTs:  Sampling time
    % iMode: Mode Selection
    % iMode=1 used as generalized 2nd-order LPF, LPF(s)=wn^2/(s^2+wn/Q*s+wn^2)
    % iMode=2 used as 2nd-order LPF in SOGI, SOGI_LPF(s)=(wn^2/Q)/(s^2+wn/Q*s+wn^2)
    % iMode=3 used as 2nd-order BPF in SOGI, SOGI_BPF(s)=(wn*s/Q)/(s^2+wn/Q*s+wn^2)
    
    persistent t;
    
    if isempty(t)
        t = zeros(2,3);
    end
    
    wn = 2*pi*fn;
    wc = wn/fQ;

    fT1 = wc*wn*fTs*fTs; 
    fT2 = 2*wc*fTs;
    fT3 = (wn*fTs)^2;
    
    fb1 = fT3+fT2+4;
    fb2 = 2*fT3-8;
    fb3 = fT3-fT2+4;
    
    if (iMode ==1)
        fa1 = fT3;
        fa2 = 2*fT3;
        fa3 = fT3;
    elseif (iMode ==2)
        fa1 = fT1;
        fa2 = 2*fT1;
        fa3 = fT1;
    else
        fa1 = fT2;
        fa2 = 0;
        fa3 = -fT2;
    end
%     if(Trigs > 0)
        t(1,1) = u;        
        t(2,1) = (fa1*t(1,1)+fa2*t(1,2)+fa3*t(1,3)-fb2*t(2,2)-fb3*t(2,3))/fb1;
    
        t(1,3) = t(1,2);
        t(1,2) = t(1,1);
        
        t(2,3) = t(2,2);
        t(2,2) = t(2,1);
%     else
%         t(1,1) = t(1,1);        
%         t(2,1) = t(2,1);
%     
%         t(1,3) = t(1,3);
%         t(1,2) = t(1,2);
%         
%         t(2,3) = t(2,3);
%         t(2,2) = t(2,2);
%     end
    
    y = t(2,1);    
end

== matlab function CSI_0313_4DC/AIP10/Subsystem5/PLL/Pos&Neg seq extract in subsystem /IIR_LPF_Im ==
  data: u input; fn input; fQ parameter; y output; fTs parameter; iMode parameter
function y =IIR_2rd(u, fn, fQ, fTs, iMode)
    % Second order transfer function used for LPF and BPF
    % y[n] = (fa1*x[n]+fa2*x[n-1]+fa3*x[n-2]-fb2*y[n-1]-fb3*y[n-2])/fb1
    % u:  error input
    % fn:  Natural frequency
    % fQ:   Quality factor
    % fTs:  Sampling time
    % iMode: Mode Selection
    % iMode=1 used as generalized 2nd-order LPF, LPF(s)=wn^2/(s^2+wn/Q*s+wn^2)
    % iMode=2 used as 2nd-order LPF in SOGI, SOGI_LPF(s)=(wn^2/Q)/(s^2+wn/Q*s+wn^2)
    % iMode=3 used as 2nd-order BPF in SOGI, SOGI_BPF(s)=(wn*s/Q)/(s^2+wn/Q*s+wn^2)
    
    persistent t;
    
    if isempty(t)
        t = zeros(2,3);
    end
    
    wn = 2*pi*fn;
    wc = wn/fQ;

    fT1 = wc*wn*fTs*fTs; 
    fT2 = 2*wc*fTs;
    fT3 = (wn*fTs)^2;
    
    fb1 = fT3+fT2+4;
    fb2 = 2*fT3-8;
    fb3 = fT3-fT2+4;
    
    if (iMode ==1)
        fa1 = fT3;
        fa2 = 2*fT3;
        fa3 = fT3;
    elseif (iMode ==2)
        fa1 = fT1;
        fa2 = 2*fT1;
        fa3 = fT1;
    else
        fa1 = fT2;
        fa2 = 0;
        fa3 = -fT2;
    end
        
%    if(Trigs > 0)
        t(1,1) = u;        
        t(2,1) = (fa1*t(1,1)+fa2*t(1,2)+fa3*t(1,3)-fb2*t(2,2)-fb3*t(2,3))/fb1;
    
        t(1,3) = t(1,2);
        t(1,2) = t(1,1);
        
        t(2,3) = t(2,2);
        t(2,2) = t(2,1);
%     else
%         t(1,1) = t(1,1);        
%         t(2,1) = t(2,1);
%     
%         t(1,3) = t(1,3);
%         t(1,2) = t(1,2);
%         
%         t(2,3) = t(2,3);
%         t(2,2) = t(2,2);
%     end
%     
    y = t(2,1);    
end

== matlab function CSI_0313_4DC/AIP8/Subsystem3/IIR_1st1 ==
  data: u input; fc parameter; y output; fTs parameter
function y = IIR_1st(u, fc, fTs)
    % y[n] = (-(1-T)*y[n-1] + x[n] + x[n-1])/(1+T)
    % u:    Input
    % fc:   Cut-off frequency
    % fTs:  Sample time
    
    persistent t;
    
    if isempty(t)
        t = zeros(2,2);
    end
    
    T = 1/(pi*fc*fTs);            
    
%     if(Trig > 0)
        t(1,1) = u;        
        t(2,1) = (t(1,1) + t(1,2) - (1-T)*t(2,2)) / (1+T);
    
        t(1,2) = t(1,1);
        t(2,2) = t(2,1);
%     else
%         t(1,1) = t(1,1);        
%         t(2,1) = t(2,1);
%     
%         t(1,2) = t(1,2);
%         t(2,2) = t(2,2);
%     end
%     
    y = t(2,1);
end

== matlab function CSI_0313_4DC/AIP8/Subsystem5/PLL/ABC_To_RIZ ==
  data: ABC input size=3; RIZ output size=3
function RIZ = ABC_To_RIZ(ABC)
    % Clarke Transfer from ABC axis to Re-Im axis
    RIZ = [0;0;0];
    RIZ(1) = (2*ABC(1)-ABC(2)-ABC(3))/3;
    RIZ(2) = sqrt(3)*(ABC(2)-ABC(3))/3;
    RIZ(3) = (ABC(1)+ABC(2)+ABC(3))/3;
end

== matlab function CSI_0313_4DC/AIP8/Subsystem5/PLL/Integral ==
  data: u input; fGain parameter; fTs parameter; y output
function y  = Integral(u, fGain, fTs)
    % y[n] = y[n-1] + (TS*0.5)*(x[n]+x[n-1])
    % u:     input
    % fGain: Gain
    % fTs:  Sampling time
    
    % t(1,2) stores x[n],x[n-1]; t(2,2) stores y[n],y[n-1]
    persistent t;      
    if isempty(t)           % Initialization
        t = zeros(2,2);
    end
%     if(Trig > 0)
        t(1,1) = u;
        t(2,1) = t(2,2) + fGain*0.5*fTs*(t(1,1)+t(1,2));   

        t(1,2) = t(1,1);
        t(2,2) = t(2,1);
%     else
%         t(1,1) = t(1,1);
%         t(2,1) = t(2,1);   
% 
%         t(1,2) = t(1,2);
%         t(2,2) = t(2,2);
%     end
    y = t(2,1);
end

== matlab function CSI_0313_4DC/AIP8/Subsystem5/PLL/PI Ctrl ==
  data: err input; y output; fKI parameter; fMinLmt parameter; fTs parameter; fMaxLmt parameter; fKP parameter
function y = PICtrl(err, fKI, fMinLmt, fTs, fMaxLmt, fKP)
    % y[n] = y[n-1] + KP*(x[n]-x[n-1]) + (KP*KI*TS*0.5)*(x[n]+x[n-1])
    % err:  error input
    % fKP:   Proportional gain
    % fKI:   Integral Coefficient
    % fMinLmt: Minimum limitation
    % fMaxLmt: Maximum limitation
    % fTs:  Sampling time
    
    % t(1,2) stores x[n],x[n-1]; t(2,2) stores y[n],y[n-1]
    persistent t;      
    if isempty(t)           % Initialization
        t = zeros(2,2);
    end

%     if(Trig > 0)
        t(1,1) = err;
        t(2,1) = t(2,2) + fKP*(t(1,1)-t(1,2)) + fKP*fKI*0.5*(t(1,1)+t(1,2))*fTs;   
    
        if (t(2,1) < fMinLmt)
            t(2,1) = fMinLmt;
        elseif (t(2,1) > fMaxLmt)
            t(2,1) = fMaxLmt;
        end
        t(1,2) = t(1,1);
        t(2,2) = t(2,1);
%     else
%         t(1,1) = t(1,1);
%         t(2,1) = t(2,1);   
%         t(1,2) = t(1,2);
%         t(2,2) = t(2,2);
%     end
    
    y = t(2,1);
end

== matlab function CSI_0313_4DC/AIP8/Subsystem5/PLL/Pos&Neg seq extract in subsystem /IIR_BPF_Im ==
  data: u input; fn input; fQ parameter; y output; fTs parameter; iMode parameter
function y =IIR_2rd(u, fn, fQ, fTs, iMode)
    % Second order transfer function used for LPF and BPF
    % y[n] = (fa1*x[n]+fa2*x[n-1]+fa3*x[n-2]-fb2*y[n-1]-fb3*y[n-2])/fb1
    % u:  error input
    % fn:  Natural frequency
    % fQ:   Quality factor
    % fTs:  Sampling time
    % iMode: Mode Selection
    % iMode=1 used as generalized 2nd-order LPF, LPF(s)=wn^2/(s^2+wn/Q*s+wn^2)
    % iMode=2 used as 2nd-order LPF in SOGI, SOGI_LPF(s)=(wn^2/Q)/(s^2+wn/Q*s+wn^2)
    % iMode=3 used as 2nd-order BPF in SOGI, SOGI_BPF(s)=(wn*s/Q)/(s^2+wn/Q*s+wn^2)
    
    persistent t;
    
    if isempty(t)
        t = zeros(2,3);
    end
    
    wn = 2*pi*fn;
    wc = wn/fQ;

    fT1 = wc*wn*fTs*fTs; 
    fT2 = 2*wc*fTs;
    fT3 = (wn*fTs)^2;
    
    fb1 = fT3+fT2+4;
    fb2 = 2*fT3-8;
    fb3 = fT3-fT2+4;
    
    if (iMode ==1)
        fa1 = fT3;
        fa2 = 2*fT3;
        fa3 = fT3;
    elseif (iMode ==2)
        fa1 = fT1;
        fa2 = 2*fT1;
        fa3 = fT1;
    else
        fa1 = fT2;
        fa2 = 0;
        fa3 = -fT2;
    end
        
%     if(Trigs > 0)
        t(1,1) = u;        
        t(2,1) = (fa1*t(1,1)+fa2*t(1,2)+fa3*t(1,3)-fb2*t(2,2)-fb3*t(2,3))/fb1;
    
        t(1,3) = t(1,2);
        t(1,2) = t(1,1);
        
        t(2,3) = t(2,2);
        t(2,2) = t(2,1);
%     else
%         t(1,1) = t(1,1);        
%         t(2,1) = t(2,1);
%     
%         t(1,3) = t(1,3);
%         t(1,2) = t(1,2);
%         
%         t(2,3) = t(2,3);
%         t(2,2) = t(2,2);
%     end
    
    y = t(2,1);    
end

== matlab function CSI_0313_4DC/AIP8/Subsystem5/PLL/Pos&Neg seq extract in subsystem /IIR_BPF_Re1 ==
  data: u input; fn input; fQ parameter; y output; fTs parameter; iMode parameter
function y =IIR_2rd(u, fn, fQ, fTs, iMode)
    % Second order transfer function used for LPF and BPF
    % y[n] = (fa1*x[n]+fa2*x[n-1]+fa3*x[n-2]-fb2*y[n-1]-fb3*y[n-2])/fb1
    % u:  error input
    % fn:  Natural frequency
    % fQ:   Quality factor
    % fTs:  Sampling time
    % iMode: Mode Selection
    % iMode=1 used as generalized 2nd-order LPF, LPF(s)=wn^2/(s^2+wn/Q*s+wn^2)
    % iMode=2 used as 2nd-order LPF in SOGI, SOGI_LPF(s)=(wn^2/Q)/(s^2+wn/Q*s+wn^2)
    % iMode=3 used as 2nd-order BPF in SOGI, SOGI_BPF(s)=(wn*s/Q)/(s^2+wn/Q*s+wn^2)
    
    persistent t;
    
    if isempty(t)
        t = zeros(2,3);
    end
    
    wn = 2*pi*fn;
    wc = wn/fQ;

    fT1 = wc*wn*fTs*fTs; 
    fT2 = 2*wc*fTs;
    fT3 = (wn*fTs)^2;
    
    fb1 = fT3+fT2+4;
    fb2 = 2*fT3-8;
    fb3 = fT3-fT2+4;
    
    if (iMode ==1)
        fa1 = fT3;
        fa2 = 2*fT3;
        fa3 = fT3;
    elseif (iMode ==2)
        fa1 = fT1;
        fa2 = 2*fT1;
        fa3 = fT1;
    else
        fa1 = fT2;
        fa2 = 0;
        fa3 = -fT2;
    end
%     if(Trigs > 0)
        t(1,1) = u;        
        t(2,1) = (fa1*t(1,1)+fa2*t(1,2)+fa3*t(1,3)-fb2*t(2,2)-fb3*t(2,3))/fb1;
    
        t(1,3) = t(1,2);
        t(1,2) = t(1,1);
        
        t(2,3) = t(2,2);
        t(2,2) = t(2,1);
%     else
%         t(1,1) = t(1,1);        
%         t(2,1) = t(2,1);
%     
%         t(1,3) = t(1,3);
%         t(1,2) = t(1,2);
%         
%         t(2,3) = t(2,3);
%         t(2,2) = t(2,2);
%     end
    
    y = t(2,1);    
end

== matlab function CSI_0313_4DC/AIP8/Subsystem5/PLL/Pos&Neg seq extract in subsystem /IIR_LPF_Im ==
  data: u input; fn input; fQ parameter; y output; fTs parameter; iMode parameter
function y =IIR_2rd(u, fn, fQ, fTs, iMode)
    % Second order transfer function used for LPF and BPF
    % y[n] = (fa1*x[n]+fa2*x[n-1]+fa3*x[n-2]-fb2*y[n-1]-fb3*y[n-2])/fb1
    % u:  error input
    % fn:  Natural frequency
    % fQ:   Quality factor
    % fTs:  Sampling time
    % iMode: Mode Selection
    % iMode=1 used as generalized 2nd-order LPF, LPF(s)=wn^2/(s^2+wn/Q*s+wn^2)
    % iMode=2 used as 2nd-order LPF in SOGI, SOGI_LPF(s)=(wn^2/Q)/(s^2+wn/Q*s+wn^2)
    % iMode=3 used as 2nd-order BPF in SOGI, SOGI_BPF(s)=(wn*s/Q)/(s^2+wn/Q*s+wn^2)
    
    persistent t;
    
    if isempty(t)
        t = zeros(2,3);
    end
    
    wn = 2*pi*fn;
    wc = wn/fQ;

    fT1 = wc*wn*fTs*fTs; 
    fT2 = 2*wc*fTs;
    fT3 = (wn*fTs)^2;
    
    fb1 = fT3+fT2+4;
    fb2 = 2*fT3-8;
    fb3 = fT3-fT2+4;
    
    if (iMode ==1)
        fa1 = fT3;
        fa2 = 2*fT3;
        fa3 = fT3;
    elseif (iMode ==2)
        fa1 = fT1;
        fa2 = 2*fT1;
        fa3 = fT1;
    else
        fa1 = fT2;
        fa2 = 0;
        fa3 = -fT2;
    end
        
%    if(Trigs > 0)
        t(1,1) = u;        
        t(2,1) = (fa1*t(1,1)+fa2*t(1,2)+fa3*t(1,3)-fb2*t(2,2)-fb3*t(2,3))/fb1;
    
        t(1,3) = t(1,2);
        t(1,2) = t(1,1);
        
        t(2,3) = t(2,2);
        t(2,2) = t(2,1);
%     else
%         t(1,1) = t(1,1);        
%         t(2,1) = t(2,1);
%     
%         t(1,3) = t(1,3);
%         t(1,2) = t(1,2);
%         
%         t(2,3) = t(2,3);
%         t(2,2) = t(2,2);
%     end
%     
    y = t(2,1);    
end

== matlab function CSI_0313_4DC/AIP8/Subsystem5/PLL/Pos&Neg seq extract in subsystem /IIR_LPF_Re1 ==
  data: u input; fn input; fQ parameter; y output; fTs parameter; iMode parameter
function y =IIR_2rd(u, fn, fQ, fTs, iMode)
    % Second order transfer function used for LPF and BPF
    % y[n] = (fa1*x[n]+fa2*x[n-1]+fa3*x[n-2]-fb2*y[n-1]-fb3*y[n-2])/fb1
    % u:  error input
    % fn:  Natural frequency
    % fQ:   Quality factor
    % fTs:  Sampling time
    % iMode: Mode Selection
    % iMode=1 used as generalized 2nd-order LPF, LPF(s)=wn^2/(s^2+wn/Q*s+wn^2)
    % iMode=2 used as 2nd-order LPF in SOGI, SOGI_LPF(s)=(wn^2/Q)/(s^2+wn/Q*s+wn^2)
    % iMode=3 used as 2nd-order BPF in SOGI, SOGI_BPF(s)=(wn*s/Q)/(s^2+wn/Q*s+wn^2)
    
    persistent t;
    
    if isempty(t)
        t = zeros(2,3);
    end
    
    wn = 2*pi*fn;
    wc = wn/fQ;

    fT1 = wc*wn*fTs*fTs; 
    fT2 = 2*wc*fTs;
    fT3 = (wn*fTs)^2;
    
    fb1 = fT3+fT2+4;
    fb2 = 2*fT3-8;
    fb3 = fT3-fT2+4;
    
    if (iMode ==1)
        fa1 = fT3;
        fa2 = 2*fT3;
        fa3 = fT3;
    elseif (iMode ==2)
        fa1 = fT1;
        fa2 = 2*fT1;
        fa3 = fT1;
    else
        fa1 = fT2;
        fa2 = 0;
        fa3 = -fT2;
    end
        
%    if(Trigs > 0)
        t(1,1) = u;        
        t(2,1) = (fa1*t(1,1)+fa2*t(1,2)+fa3*t(1,3)-fb2*t(2,2)-fb3*t(2,3))/fb1;
    
        t(1,3) = t(1,2);
        t(1,2) = t(1,1);
        
        t(2,3) = t(2,2);
        t(2,2) = t(2,1);
%     else
%         t(1,1) = t(1,1);        
%         t(2,1) = t(2,1);
%     
%         t(1,3) = t(1,3);
%         t(1,2) = t(1,2);
%         
%         t(2,3) = t(2,3);
%         t(2,2) = t(2,2);
%     end
    
    y = t(2,1);    
end

== matlab function CSI_0313_4DC/AIP8/Subsystem5/PLL/RIZ_To_DQ0 ==
  data: RIZ input; DQ0 output; wt input; iAxis parameter
function DQ0 = RIZ_To_DQ0(RIZ,wt,iAxis)
    % Park Transfer from Re-Im axis to DQ0 axis
    DQ0 = [0;0;0];
    if (iAxis == 1)
        DQ0(1) = RIZ(1)*cos(wt)+RIZ(2)*sin(wt);
        DQ0(2) = -RIZ(1)*sin(wt)+RIZ(2)*cos(wt);
    else
        DQ0(1) = RIZ(1)*sin(wt)-RIZ(2)*cos(wt);
        DQ0(2) = RIZ(1)*cos(wt)+RIZ(2)*sin(wt);
    end
end

== matlab function CSI_0313_4DC/AIP8/Subsystem7/ABC_To_RIZ1 ==
  data: ABC input; RIZ output
function RIZ = ABC_To_RIZ(ABC)
    % Clarke Transfer from ABC axis to Re-Im axis
    RIZ = [0;0;0];
    RIZ(1) = (2*ABC(1)-ABC(2)-ABC(3))/3;
    RIZ(2) = sqrt(3)*(ABC(2)-ABC(3))/3;
    RIZ(3) = (ABC(1)+ABC(2)+ABC(3))/3;
end

== matlab function CSI_0313_4DC/AIP8/Subsystem7/BPF /IIR_BPF_Re1 ==
  data: u input; fn input; fQ parameter; y output; fTs parameter; iMode parameter
function y =IIR_2rd(u, fn, fQ, fTs, iMode)
    % Second order transfer function used for LPF and BPF
    % y[n] = (fa1*x[n]+fa2*x[n-1]+fa3*x[n-2]-fb2*y[n-1]-fb3*y[n-2])/fb1
    % u:  error input
    % fn:  Natural frequency
    % fQ:   Quality factor
    % fTs:  Sampling time
    % iMode: Mode Selection
    % iMode=1 used as generalized 2nd-order LPF, LPF(s)=wn^2/(s^2+wn/Q*s+wn^2)
    % iMode=2 used as 2nd-order LPF in SOGI, SOGI_LPF(s)=(wn^2/Q)/(s^2+wn/Q*s+wn^2)
    % iMode=3 used as 2nd-order BPF in SOGI, SOGI_BPF(s)=(wn*s/Q)/(s^2+wn/Q*s+wn^2)
    
    persistent t;
    
    if isempty(t)
        t = zeros(2,3);
    end
    
    wn = 2*pi*fn;
    wc = wn/fQ;

    fT1 = wc*wn*fTs*fTs; 
    fT2 = 2*wc*fTs;
    fT3 = (wn*fTs)^2;
    
    fb1 = fT3+fT2+4;
    fb2 = 2*fT3-8;
    fb3 = fT3-fT2+4;
    
    if (iMode ==1)
        fa1 = fT3;
        fa2 = 2*fT3;
        fa3 = fT3;
    elseif (iMode ==2)
        fa1 = fT1;
        fa2 = 2*fT1;
        fa3 = fT1;
    else
        fa1 = fT2;
        fa2 = 0;
        fa3 = -fT2;
    end
 
        t(1,1) = u;        
        t(2,1) = (fa1*t(1,1)+fa2*t(1,2)+fa3*t(1,3)-fb2*t(2,2)-fb3*t(2,3))/fb1;
    
        t(1,3) = t(1,2);
        t(1,2) = t(1,1);
        
        t(2,3) = t(2,2);
        t(2,2) = t(2,1);
 
    
    y = t(2,1);    
end

== matlab function CSI_0313_4DC/AIP8/Subsystem7/BPF /IIR_BPF_Re2 ==
  data: u input; fn input; fQ parameter; y output; fTs parameter; iMode parameter
function y =IIR_2rd(u, fn, fQ, fTs, iMode)
    % Second order transfer function used for LPF and BPF
    % y[n] = (fa1*x[n]+fa2*x[n-1]+fa3*x[n-2]-fb2*y[n-1]-fb3*y[n-2])/fb1
    % u:  error input
    % fn:  Natural frequency
    % fQ:   Quality factor
    % fTs:  Sampling time
    % iMode: Mode Selection
    % iMode=1 used as generalized 2nd-order LPF, LPF(s)=wn^2/(s^2+wn/Q*s+wn^2)
    % iMode=2 used as 2nd-order LPF in SOGI, SOGI_LPF(s)=(wn^2/Q)/(s^2+wn/Q*s+wn^2)
    % iMode=3 used as 2nd-order BPF in SOGI, SOGI_BPF(s)=(wn*s/Q)/(s^2+wn/Q*s+wn^2)
    
    persistent t;
    
    if isempty(t)
        t = zeros(2,3);
    end
    
    wn = 2*pi*fn;
    wc = wn/fQ;

    fT1 = wc*wn*fTs*fTs; 
    fT2 = 2*wc*fTs;
    fT3 = (wn*fTs)^2;
    
    fb1 = fT3+fT2+4;
    fb2 = 2*fT3-8;
    fb3 = fT3-fT2+4;
    
    if (iMode ==1)
        fa1 = fT3;
        fa2 = 2*fT3;
        fa3 = fT3;
    elseif (iMode ==2)
        fa1 = fT1;
        fa2 = 2*fT1;
        fa3 = fT1;
    else
        fa1 = fT2;
        fa2 = 0;
        fa3 = -fT2;
    end
  
        t(1,1) = u;        
        t(2,1) = (fa1*t(1,1)+fa2*t(1,2)+fa3*t(1,3)-fb2*t(2,2)-fb3*t(2,3))/fb1;
    
        t(1,3) = t(1,2);
        t(1,2) = t(1,1);
        
        t(2,3) = t(2,2);
        t(2,2) = t(2,1);
 
    
    y = t(2,1);    
end

== matlab function CSI_0313_4DC/AIP8/Subsystem7/BPF /IIR_BPF_Re3 ==
  data: u input; fn input; fQ parameter; y output; fTs parameter; iMode parameter
function y =IIR_2rd(u, fn, fQ, fTs, iMode)
    % Second order transfer function used for LPF and BPF
    % y[n] = (fa1*x[n]+fa2*x[n-1]+fa3*x[n-2]-fb2*y[n-1]-fb3*y[n-2])/fb1
    % u:  error input
    % fn:  Natural frequency
    % fQ:   Quality factor
    % fTs:  Sampling time
    % iMode: Mode Selection
    % iMode=1 used as generalized 2nd-order LPF, LPF(s)=wn^2/(s^2+wn/Q*s+wn^2)
    % iMode=2 used as 2nd-order LPF in SOGI, SOGI_LPF(s)=(wn^2/Q)/(s^2+wn/Q*s+wn^2)
    % iMode=3 used as 2nd-order BPF in SOGI, SOGI_BPF(s)=(wn*s/Q)/(s^2+wn/Q*s+wn^2)
    
    persistent t;
    
    if isempty(t)
        t = zeros(2,3);
    end
    
    wn = 2*pi*fn;
    wc = wn/fQ;

    fT1 = wc*wn*fTs*fTs; 
    fT2 = 2*wc*fTs;
    fT3 = (wn*fTs)^2;
    
    fb1 = fT3+fT2+4;
    fb2 = 2*fT3-8;
    fb3 = fT3-fT2+4;
    
    if (iMode ==1)
        fa1 = fT3;
        fa2 = 2*fT3;
        fa3 = fT3;
    elseif (iMode ==2)
        fa1 = fT1;
        fa2 = 2*fT1;
        fa3 = fT1;
    else
        fa1 = fT2;
        fa2 = 0;
        fa3 = -fT2;
    end
  
        t(1,1) = u;        
        t(2,1) = (fa1*t(1,1)+fa2*t(1,2)+fa3*t(1,3)-fb2*t(2,2)-fb3*t(2,3))/fb1;
    
        t(1,3) = t(1,2);
        t(1,2) = t(1,1);
        
        t(2,3) = t(2,2);
        t(2,2) = t(2,1);
 
    
    y = t(2,1);    
end

== matlab function CSI_0313_4DC/AIP8/Subsystem7/Pos Compensation1/DQ0_To_RIZ ==
  data: DQ0 input; RIZ output; wt input; iAxis parameter
function RIZ = DQ0_To_RIZ(DQ0,wt,iAxis)
    % Inverse Park Transfer from DQ0 axis to Re-Im axis
    RIZ = [0;0;0];
    if (iAxis == 1)
        RIZ(1) = DQ0(1)*cos(wt)-DQ0(2)*sin(wt);
        RIZ(2) = DQ0(1)*sin(wt)+DQ0(2)*cos(wt);
    else
        RIZ(1) = DQ0(1)*sin(wt)+DQ0(2)*cos(wt);
        RIZ(2) = -DQ0(1)*cos(wt)+DQ0(2)*sin(wt);
    end
end

== matlab function CSI_0313_4DC/AIP10/Subsystem5/PLL/Pos&Neg seq extract in subsystem /IIR_LPF_Re1 ==
  data: u input; fn input; fQ parameter; y output; fTs parameter; iMode parameter
function y =IIR_2rd(u, fn, fQ, fTs, iMode)
    % Second order transfer function used for LPF and BPF
    % y[n] = (fa1*x[n]+fa2*x[n-1]+fa3*x[n-2]-fb2*y[n-1]-fb3*y[n-2])/fb1
    % u:  error input
    % fn:  Natural frequency
    % fQ:   Quality factor
    % fTs:  Sampling time
    % iMode: Mode Selection
    % iMode=1 used as generalized 2nd-order LPF, LPF(s)=wn^2/(s^2+wn/Q*s+wn^2)
    % iMode=2 used as 2nd-order LPF in SOGI, SOGI_LPF(s)=(wn^2/Q)/(s^2+wn/Q*s+wn^2)
    % iMode=3 used as 2nd-order BPF in SOGI, SOGI_BPF(s)=(wn*s/Q)/(s^2+wn/Q*s+wn^2)
    
    persistent t;
    
    if isempty(t)
        t = zeros(2,3);
    end
    
    wn = 2*pi*fn;
    wc = wn/fQ;

    fT1 = wc*wn*fTs*fTs; 
    fT2 = 2*wc*fTs;
    fT3 = (wn*fTs)^2;
    
    fb1 = fT3+fT2+4;
    fb2 = 2*fT3-8;
    fb3 = fT3-fT2+4;
    
    if (iMode ==1)
        fa1 = fT3;
        fa2 = 2*fT3;
        fa3 = fT3;
    elseif (iMode ==2)
        fa1 = fT1;
        fa2 = 2*fT1;
        fa3 = fT1;
    else
        fa1 = fT2;
        fa2 = 0;
        fa3 = -fT2;
    end
        
%    if(Trigs > 0)
        t(1,1) = u;        
        t(2,1) = (fa1*t(1,1)+fa2*t(1,2)+fa3*t(1,3)-fb2*t(2,2)-fb3*t(2,3))/fb1;
    
        t(1,3) = t(1,2);
        t(1,2) = t(1,1);
        
        t(2,3) = t(2,2);
        t(2,2) = t(2,1);
%     else
%         t(1,1) = t(1,1);        
%         t(2,1) = t(2,1);
%     
%         t(1,3) = t(1,3);
%         t(1,2) = t(1,2);
%         
%         t(2,3) = t(2,3);
%         t(2,2) = t(2,2);
%     end
    
    y = t(2,1);    
end

== matlab function CSI_0313_4DC/AIP8/Subsystem7/Pos Compensation1/RIZ_To_ABC ==
  data: RIZ input; ABC output
function ABC = RIZ_To_ABC(RIZ)
    % Inverse Clarke Transfer from Re-Im axis to ABC axis
    ABC = [0;0;0];
    ABC(1) = RIZ(1)+RIZ(3);
    ABC(2) = -(RIZ(1)-sqrt(3)*RIZ(2))/2+RIZ(3);
    ABC(3) = -(RIZ(1)+sqrt(3)*RIZ(2))/2+RIZ(3);
end

== matlab function CSI_0313_4DC/AIP8/Subsystem7/Pos Compensation1/RIZ_To_DQ0 ==
  data: RIZ input; DQ0 output; wt input; iAxis parameter
function DQ0 = RIZ_To_DQ0(RIZ,wt,iAxis)
    % Park Transfer from Re-Im axis to DQ0 axis
    DQ0 = [0;0;0];
    if (iAxis == 1)
        DQ0(1) = RIZ(1)*cos(wt)+RIZ(2)*sin(wt);
        DQ0(2) = -RIZ(1)*sin(wt)+RIZ(2)*cos(wt);
    else
        DQ0(1) = RIZ(1)*sin(wt)-RIZ(2)*cos(wt);
        DQ0(2) = RIZ(1)*cos(wt)+RIZ(2)*sin(wt);
    end
end

== matlab function CSI_0313_4DC/AIP8/Subsystem7/RIZ_To_ABC1 ==
  data: RIZ input; ABC output
function ABC = RIZ_To_ABC(RIZ)
    % Inverse Clarke Transfer from Re-Im axis to ABC axis
    ABC = [0;0;0];
    ABC(1) = RIZ(1)+RIZ(3);
    ABC(2) = -(RIZ(1)-sqrt(3)*RIZ(2))/2+RIZ(3);
    ABC(3) = -(RIZ(1)+sqrt(3)*RIZ(2))/2+RIZ(3);
end

== matlab function CSI_0313_4DC/AIP8/Subsystem7/Subsystem5/3rd Injection1 ==
  data: Vabc input; Mod output size=3; Vdc input; mode parameter
function Mod = fcn(Vabc,Vdc,mode)

Mod = Vabc./(Vdc/2);
Vmin = min(Mod(1),min(Mod(2),Mod(3)));
Vmax = max(Mod(1),max(Mod(2),Mod(3)));
Vinj= -0.5*(Vmin+Vmax);
if(mode == 0)
    Mod(1) = Mod(1)+Vinj;
    Mod(2) = Mod(2)+Vinj;
    Mod(3) = Mod(3)+Vinj;
else
    Mod(1) = Mod(1);
    Mod(2) = Mod(2);
    Mod(3) = Mod(3);    
end
end

function y = min(a,b)
    if (a <= b)
        y = a;
    else
        y = b;
    end
end

function y = max(a,b)
    if (a >= b)
        y = a;
    else
        y = b;
    end
end

== matlab function CSI_0313_4DC/AIP8/VLine_To_VPh ==
  data: VLine input; VPh output
function VPh = VLine_To_VPh(VLine)
    % Assume Van+Vbn+Vcn=0
    % VLine(1)=Vab; VLine(2)=Vbc; VLine(3)=Vca 
    % VPh(1)=Van; VPh(2)=Vbn; VPh(3)=Vcn;
    VPh = [0;0;0];
    VPh(1) = (VLine(1)-VLine(3))/3;
    VPh(2) = (VLine(2)-VLine(1))/3;
    VPh(3) = (VLine(3)-VLine(2))/3;
end
